simulink model "modelo"  (R2020b)
settings: Solver=VariableStepAuto  StartTime=0.0  StopTime=10.0  FixedStep=1e-3  RelTol=1e-3
undefined symbols (not defined in the file): den1, den2, den3, k, num1, num2, num3
settings Model: Creator=Aitor  LastModifiedBy=Aitor

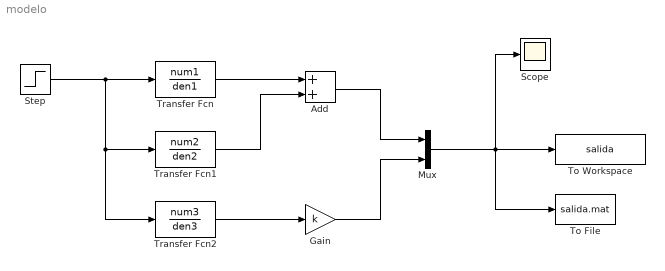
== system modelo ==
  Add : Sum
  Gain : Gain  Gain=k
  Mux : Mux  Inputs=2
  Scope : Scope
  Step : Step  Time=0.5  After=2  SampleTime=0
  To File : ToFile  Filename=salida.mat
  To Workspace : ToWorkspace  VariableName=salida  SaveFormat=Timeseries  SampleTime=-1
  Transfer Fcn : TransferFcn  Numerator=num1  Denominator=den1
  Transfer Fcn1 : TransferFcn  Numerator=num2  Denominator=den2
  Transfer Fcn2 : TransferFcn  Numerator=num3  Denominator=den3
  wires:
  Step/1 -> Transfer Fcn2/1, Transfer Fcn1/1, Transfer Fcn/1
  Transfer Fcn/1 -> Add/1
  Transfer Fcn1/1 -> Add/2
  Transfer Fcn2/1 -> Gain/1
  Add/1 -> Mux/1
  Gain/1 -> Mux/2
  Mux/1 -> Scope/1, To File/1, To Workspace/1
